simulink library "Tire_MFSwift"  (R2026a)
settings: Solver=VariableStepAuto
undefined symbols (not defined in the file): Left, mfswift_Veh_PARAM, Vehicle, Visual, X, Y, Z
libraries: nesl_utility x24, sm_lib x15, TireBody_Systems x1, mfswift_library x1, mfswift_simscape_library x1, Tire_Utilities x1, $bdroot x1
(part 2 of 2)

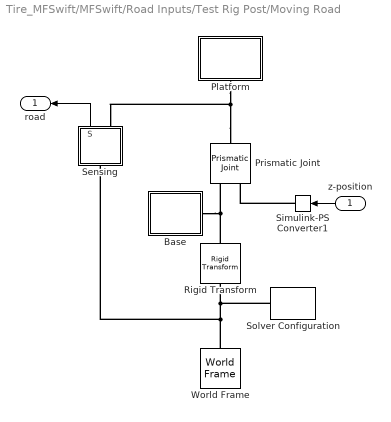
== system Tire_MFSwift/MFSwift/Road Inputs/Test Rig Post/Moving Road ==
  z-position : Inport
  Base : Subsystem
  Platform : Subsystem
  Prismatic Joint : sm_lib/Joints/Prismatic Joint  JointMode=Normal  CompositeWrenchDir=FollowerOnBase  CompositeWrenchFrame=BaseFrame  SenseConstraintForce=off  SenseConstraintTorque=off  SenseTotalForce=off  SenseTotalTorque=off  PositionTargetSpecify=off  PositionTargetPriority=High  PositionTargetValue=0  PositionTargetValueUnits=m  VelocityTargetSpecify=off  VelocityTargetPriority=High  VelocityTargetValue=0  VelocityTargetValueUnits=m/s  EquilibriumPosition=0  EquilibriumPositionUnits=m  SpringStiffness=0  SpringStiffnessUnits=N/m  DampingCoefficient=0  DampingCoefficientUnits=N/(m/s)  LowerLimitSpecify=off  LowerLimitBound=-1  LowerLimitBoundUnits=m  LowerLimitStiffness=1e6  LowerLimitStiffnessUnits=N/m  LowerLimitDamping=1e3  LowerLimitDampingUnits=N/(m/s)  LowerLimitTransitionRegionWidth=1e-4  LowerLimitTransitionRegionWidthUnits=m  UpperLimitSpecify=off  UpperLimitBound=1  UpperLimitBoundUnits=m  UpperLimitStiffness=1e6  UpperLimitStiffnessUnits=N/m  UpperLimitDamping=1e3  UpperLimitDampingUnits=N/(m/s)  UpperLimitTransitionRegionWidth=1e-4  UpperLimitTransitionRegionWidthUnits=m  TorqueActuationMode=ComputedTorque  MotionActuationMode=InputMotion  SensePosition=off  SenseVelocity=off  SenseAcceleration=off  SenseTorqueForce=off  SenseLowerLimitTorqueForce=off  SenseUpperLimitTorqueForce=off
  Rigid Transform : sm_lib/Frames and Transforms/Rigid Transform  RotationMethod=None  FollAlignAxisA=+X  BaseAlignAxisA=+Y  FollAlignAxisB=+Y  BaseAlignAxisB=+Z  RotationStandardAxis=+X  RotationAngle=0  RotationAngleUnits=deg  RotationArbitraryAxis=[0 0 1]  RotationSequenceAxes=FollowerAxes  RotationSequence=XYX  RotationSequenceAngles=[0 0 0]  RotationSequenceAnglesUnits=deg  RotationMatrix=[1 0 0; 0 1 0; 0 0 1]  Quaternion=[1 0 0 0]  TranslationMethod=Cartesian  TranslationCartesianOffset=[mfswift_Veh_PARAM.Body.Length*frontrear mfswift_Veh_PARAM.WheelBase/2*leftright 0]  TranslationCartesianOffsetUnits=m  TranslationStandardAxis=+Z  TranslationStandardOffset=0  TranslationStandardOffsetUnits=m  TranslationROffset=0  TranslationROffsetUnits=m  TranslationThetaOffset=0  TranslationThetaOffsetUnits=deg  TranslationZOffset=0  TranslationZOffsetUnits=m
  Sensing : Subsystem
  Simulink-PS Converter1 : nesl_utility/Simulink-PS Converter  PhysicalDomain=network_engine_domain  SubClassName=ps_input  LeftPortType=input  RightPortType=output  PseudoPeriodic=off  Frequencies=[]  NoiseDistribution=none  NoiseParameters=[]  Unit=1  AffineConversion=off  FilteringAndDerivatives=zero  SimscapeFilterOrder=2  InputFilterTimeConstant=response_time*0.1075  UdotUserProvided=1
  Solver Configuration : nesl_utility/Solver Configuration  PhysicalDomain=network_engine_domain  SubClassName=solver  LeftPortType=input  RightPortType=generic  Tones=[]  Harmonics=[]  SimulateNoise=off  Profile=off  UseLocalSampling=off  EnableSwitchedLinearOptims=on  FrequencyDomain=off  UseCCode=off  RelTol=0.001  AbsTol=1e-06  MinStep=1e-09  ToWorkspace=off  RevertToSquareIcSolve=off  NumHomotopyIterations=100  PhasorMode=off  PhasorModeNumHarmonics=1  ConsistencySolver=NEWTON_FTOL  CanonicalOrdering=UNORDERED  OptimizeIntermediates=UNOPTIMIZED  IndexReductionMethod=DerivativeReplacement  DoDC=off  ResidualTolerance=1e-09  ConsistencyTolSource=GLOBAL  ConsistencyAbsTol=0.001  ConsistencyRelTol=0.001  ConsistencyTolFactor=0.001  UseLocalSolver=off  LocalSolverChoice=NE_BACKWARD_EULER_ADVANCER  ResolveIndetEquations=on  FunctionEvalNumThread=1  LocalSolverSampleTime=0.001  DoFixedCost=off  MaxNonlinIter=3  MaxModeIter=2  ComputeImpulses=off  ImpulseIterations=2  LinearAlgebra=Sparse  LinearAlgebraNumThread=0  EquationFormulation=NE_TIME_EF  DelaysMemoryBudget=1024  AutomaticFiltering=on  FilteringTimeConstant=0.001  PartitionStorageMethod=AS_NEEDED  PartitionMemoryBudget=1024  PartitionMethod=FAST  MultibodyUseLocalSolver=off  MultibodyLocalSolverChoice=ODE1  MultibodyLocalSolverSampleTime=0.001
  World Frame : sm_lib/Frames and Transforms/World Frame
  road : Outport
  wires:
  Sensing/1(S) -> road/1
  z-position/1 -> Simulink-PS Converter1/1
  connections:
  Prismatic Joint/RConn1 -- Sensing/RConn1 -- Platform/LConn1
  Prismatic Joint/LConn1 -- Base/RConn1 -- Rigid Transform/RConn1
  Sensing/LConn1 -- Solver Configuration/RConn1 -- Rigid Transform/LConn1 -- World Frame/RConn1
  Simulink-PS Converter1/RConn1 -- Prismatic Joint/LConn2

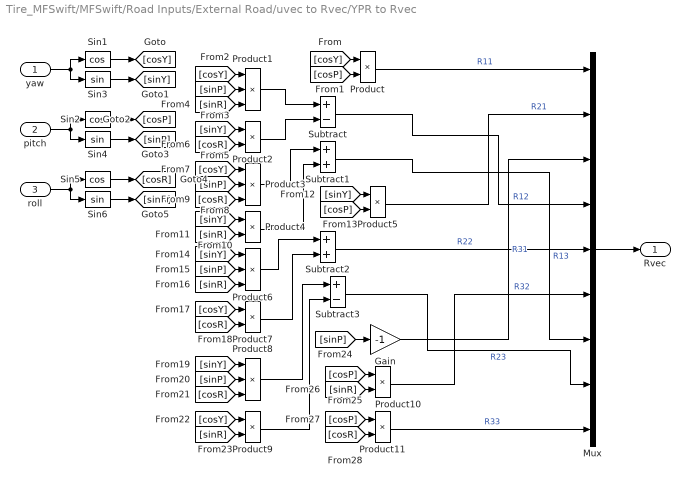
== system Tire_MFSwift/MFSwift/Road Inputs/External Road/uvec to Rvec/YPR to Rvec ==
  yaw : Inport
  pitch : Inport  Port=2
  roll : Inport  Port=3
  Gain : Gain  Gain=-1
  Mux : Mux  Inputs=9
  Product{,2,4..5,7,9..11} (8 alike) : Product
  Product{1,3,6,8} (4 alike) : Product  Inputs=3
  Sin1 : Trigonometry  Operator=cos
  Sin2 : Trigonometry  Operator=cos
  Sin3 : Trigonometry
  Sin4 : Trigonometry
  Sin5 : Trigonometry  Operator=cos
  Sin6 : Trigonometry
  Subtract : Sum  Inputs=+-
  Subtract1 : Sum
  Subtract2 : Sum
  Subtract3 : Sum  Inputs=+-
  Rvec : Outport
  wires:
  Sin4/1 -> [sinP]
  [sinP] -> Product6/2
  Product4/1 -> Subtract1/2
  [cosY] -> Product3/1
  Subtract3/1 -> Mux/8  "R23"
  [sinY] -> Product8/1
  Subtract2/1 -> Mux/5  "R22"
  [cosP] -> Product10/1
  [cosY] -> Product/1
  [sinP] -> Product3/2
  [sinY] -> Product2/1
  yaw/1 -> Sin1/1, Sin3/1
  Subtract/1 -> Mux/4  "R12"
  Sin2/1 -> [cosP]
  Sin5/1 -> [cosR]
  [cosR] -> Product11/2
  [sinP] -> Gain/1
  [sinR] -> Product10/2
  [sinR] -> Product1/3
  [cosR] -> Product8/3
  roll/1 -> Sin5/1, Sin6/1
  Product5/1 -> Mux/2  "R21"
  Product8/1 -> Subtract3/1
  Sin1/1 -> [cosY]
  [cosR] -> Product7/2
  Product11/1 -> Mux/9  "R33"
  Product1/1 -> Subtract/1
  [sinY] -> Product4/1
  [sinP] -> Product8/2
  [cosY] -> Product1/1
  [cosY] -> Product7/1
  Sin6/1 -> [sinR]
  Product2/1 -> Subtract/2
  [cosY] -> Product9/1
  [cosP] -> Product11/1
  [cosP] -> Product/2
  Product9/1 -> Subtract3/2
  [cosR] -> Product2/2
  [sinR] -> Product4/2
  Product/1 -> Mux/1  "R11"
  [sinY] -> Product5/1
  Product7/1 -> Subtract2/2
  [cosP] -> Product5/2
  Sin3/1 -> [sinY]
  Product10/1 -> Mux/6  "R32"
  [sinP] -> Product1/2
  [cosR] -> Product3/3
  Gain/1 -> Mux/3  "R31"
  Mux/1 -> Rvec/1
  pitch/1 -> Sin4/1, Sin2/1
  [sinY] -> Product6/1
  Subtract1/1 -> Mux/7  "R13"
  Product6/1 -> Subtract2/1
  [sinR] -> Product6/3
  [sinR] -> Product9/2
  Product3/1 -> Subtract1/1

== system Tire_MFSwift/MFSwift/Road Inputs/Test Rig Post/Moving Road/Base ==
  Platform1 : sm_lib/Body Elements/Cylindrical Solid  CylinderRadius=0.15  CylinderRadiusUnits=m  CylinderLength=0.5  CylinderLengthUnits=m  ExportEntireGeometry=off  InertiaType=CalculateFromGeometry  BasedOnType=Density  Density=1000  DensityUnits=kg/(m^3)  Mass=1  MassUnits=kg  CenterOfMass=[0 0 0]  CenterOfMassUnits=m  MomentsOfInertia=[1 1 1]  MomentsOfInertiaUnits=kg*m^2  ProductsOfInertia=[0 0 0]  ProductsOfInertiaUnits=kg*m^2  GraphicType=FromGeometry  MarkerShape=Sphere  MarkerSize=10  GraphicVisPropType=SimpleVisualProperties  GraphicDiffuseColor=[0.5 0.5 0.5]  GraphicOpacity=0.5  GraphicSpecularColor=[0.5 0.5 0.5 1.0]  GraphicAmbientColor=[0.15 0.15 0.15 1.0]  GraphicEmissiveColor=[0.0 0.0 0.0 1.0]  GraphicShininess=75  DoExposeReferenceFrame=on  SerializedFrames=<Frames/>
  Rigid Transform1 : sm_lib/Frames and Transforms/Rigid Transform  RotationMethod=None  FollAlignAxisA=+X  BaseAlignAxisA=+Y  FollAlignAxisB=+Y  BaseAlignAxisB=+Z  RotationStandardAxis=+Z  RotationAngle=0  RotationAngleUnits=deg  RotationArbitraryAxis=[0 0 1]  RotationSequenceAxes=FollowerAxes  RotationSequence=XYX  RotationSequenceAngles=[0 0 0]  RotationSequenceAnglesUnits=deg  RotationMatrix=[1 0 0; 0 1 0; 0 0 1]  Quaternion=[1 0 0 0]  TranslationMethod=Cartesian  TranslationCartesianOffset=[0 0 -0.50]  TranslationCartesianOffsetUnits=m  TranslationStandardAxis=+Z  TranslationStandardOffset=0  TranslationStandardOffsetUnits=m  TranslationROffset=0  TranslationROffsetUnits=m  TranslationThetaOffset=0  TranslationThetaOffsetUnits=deg  TranslationZOffset=0  TranslationZOffsetUnits=m
  B : PMIOPort  Side=Right
  connections:
  Rigid Transform1/RConn1 -- Platform1/RConn1
  Rigid Transform1/LConn1 -- B/RConn1

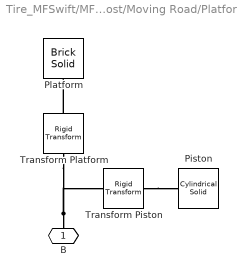
== system Tire_MFSwift/MFSwift/Road Inputs/Test Rig Post/Moving Road/Platform ==
  Piston : sm_lib/Body Elements/Cylindrical Solid  CylinderRadius=0.07  CylinderRadiusUnits=m  CylinderLength=0.4  CylinderLengthUnits=m  ExportEntireGeometry=off  InertiaType=CalculateFromGeometry  BasedOnType=Density  Density=1000  DensityUnits=kg/(m^3)  Mass=1  MassUnits=kg  CenterOfMass=[0 0 0]  CenterOfMassUnits=m  MomentsOfInertia=[1 1 1]  MomentsOfInertiaUnits=kg*m^2  ProductsOfInertia=[0 0 0]  ProductsOfInertiaUnits=kg*m^2  GraphicType=FromGeometry  MarkerShape=Sphere  MarkerSize=10  GraphicVisPropType=SimpleVisualProperties  GraphicDiffuseColor=[0.8 0.8 0.8]  GraphicOpacity=1.0  GraphicSpecularColor=[0.5 0.5 0.5 1.0]  GraphicAmbientColor=[0.15 0.15 0.15 1.0]  GraphicEmissiveColor=[0.0 0.0 0.0 1.0]  GraphicShininess=75  DoExposeReferenceFrame=on  SerializedFrames=<Frames/>
  Platform : sm_lib/Body Elements/Brick Solid  BrickDimensions=[0.5 0.5 0.04]  BrickDimensionsUnits=m  ExportEntireGeometry=off  InertiaType=CalculateFromGeometry  BasedOnType=Density  Density=1000  DensityUnits=kg/(m^3)  Mass=1  MassUnits=kg  CenterOfMass=[0 0 0]  CenterOfMassUnits=m  MomentsOfInertia=[1 1 1]  MomentsOfInertiaUnits=kg*m^2  ProductsOfInertia=[0 0 0]  ProductsOfInertiaUnits=kg*m^2  GraphicType=FromGeometry  MarkerShape=Sphere  MarkerSize=10  GraphicVisPropType=SimpleVisualProperties  GraphicDiffuseColor=[0.5 0.5 0.5]  GraphicOpacity=1.0  GraphicSpecularColor=[0.5 0.5 0.5 1.0]  GraphicAmbientColor=[0.15 0.15 0.15 1.0]  GraphicEmissiveColor=[0.0 0.0 0.0 1.0]  GraphicShininess=75  DoExposeReferenceFrame=on  SerializedFrames=<Frames/>
  Transform Piston : sm_lib/Frames and Transforms/Rigid Transform  RotationMethod=None  FollAlignAxisA=+X  BaseAlignAxisA=+Y  FollAlignAxisB=+Y  BaseAlignAxisB=+Z  RotationStandardAxis=+Z  RotationAngle=0  RotationAngleUnits=deg  RotationArbitraryAxis=[0 0 1]  RotationSequenceAxes=FollowerAxes  RotationSequence=XYX  RotationSequenceAngles=[0 0 0]  RotationSequenceAnglesUnits=deg  RotationMatrix=[1 0 0; 0 1 0; 0 0 1]  Quaternion=[1 0 0 0]  TranslationMethod=Cartesian  TranslationCartesianOffset=[0 0 -0.26]  TranslationCartesianOffsetUnits=m  TranslationStandardAxis=+Z  TranslationStandardOffset=0  TranslationStandardOffsetUnits=m  TranslationROffset=0  TranslationROffsetUnits=m  TranslationThetaOffset=0  TranslationThetaOffsetUnits=deg  TranslationZOffset=0  TranslationZOffsetUnits=m
  Transform Platform : sm_lib/Frames and Transforms/Rigid Transform  RotationMethod=None  FollAlignAxisA=+X  BaseAlignAxisA=+Y  FollAlignAxisB=+Y  BaseAlignAxisB=+Z  RotationStandardAxis=+Z  RotationAngle=0  RotationAngleUnits=deg  RotationArbitraryAxis=[0 0 1]  RotationSequenceAxes=FollowerAxes  RotationSequence=XYX  RotationSequenceAngles=[0 0 0]  RotationSequenceAnglesUnits=deg  RotationMatrix=[1 0 0; 0 1 0; 0 0 1]  Quaternion=[1 0 0 0]  TranslationMethod=Cartesian  TranslationCartesianOffset=[0 0 -0.06]  TranslationCartesianOffsetUnits=m  TranslationStandardAxis=+Z  TranslationStandardOffset=0  TranslationStandardOffsetUnits=m  TranslationROffset=0  TranslationROffsetUnits=m  TranslationThetaOffset=0  TranslationThetaOffsetUnits=deg  TranslationZOffset=0  TranslationZOffsetUnits=m
  B : PMIOPort  Side=Left
  connections:
  B/RConn1 -- Transform Piston/LConn1 -- Transform Platform/LConn1
  Transform Platform/RConn1 -- Platform/RConn1
  Transform Piston/RConn1 -- Piston/RConn1

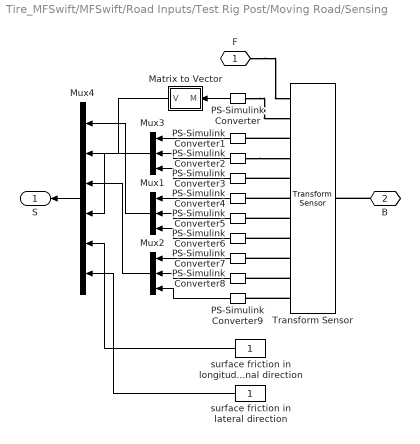
== system Tire_MFSwift/MFSwift/Road Inputs/Test Rig Post/Moving Road/Sensing ==
  Matrix to Vector : Subsystem
  Mux1 : Mux  Inputs=3
  Mux2 : Mux  Inputs=3
  Mux3 : Mux  Inputs=3
  Mux4 : Mux  Inputs=6
  PS-Simulink Converter{,1..9} (10 alike) : nesl_utility/PS-Simulink Converter  PhysicalDomain=network_engine_domain  SubClassName=ps_output  LeftPortType=input  RightPortType=output  PseudoPeriodic=off  Frequencies=[]  VectorFormat=1-D array  Unit=1  AffineConversion=off
  Transform Sensor : sm_lib/Frames and Transforms/Transform Sensor  MeasurementFrame=World  RotationSequence=XYX  SenseAngle=off  SenseAxis=off  SenseQ=off  SenseR=on  SenseRotationSequence=off  SenseOmegaX=on  SenseOmegaY=on  SenseOmegaZ=on  SenseOmega=off  SenseQDot=off  SenseRDot=off  SenseRotationSequenceDot=off  SenseAlphaX=off  SenseAlphaY=off  SenseAlphaZ=off  SenseAlpha=off  SenseQDDot=off  SenseRDDot=off  SenseX=on  SenseY=on  SenseZ=on  SenseXYZ=off  SenseRad=off  SenseAzim=off  SenseDist=off  SenseInc=off  SenseXDot=on  SenseYDot=on  SenseZDot=on  SenseXYZDot=off  SenseRadDot=off  SenseAzimDot=off  SenseDistDot=off  SenseIncDot=off  SenseXDDot=off  SenseYDDot=off  SenseZDDot=off  SenseXYZDDot=off  SenseRadDDot=off  SenseAzimDDot=off  SenseDistDDot=off  SenseIncDDot=off
  surface friction in lateral direction : Constant
  surface friction in longitudinal direction : Constant
  F : PMIOPort  Side=Right
  B : PMIOPort  Port=2  Side=Left
  S : Outport
  wires:
  surface friction in lateral direction/1 -> Mux4/6
  surface friction in longitudinal direction/1 -> Mux4/5
  Matrix to Vector/1(V) -> Mux4/2
  PS-Simulink Converter8/1 -> Mux2/2
  PS-Simulink Converter1/1 -> Mux3/1
  Mux3/1 -> Mux4/4
  PS-Simulink Converter9/1 -> Mux2/3
  Mux1/1 -> Mux4/1
  Mux2/1 -> Mux4/3
  Mux4/1 -> S/1
  PS-Simulink Converter3/1 -> Mux3/3
  PS-Simulink Converter/1 -> Matrix to Vector/1(M)
  PS-Simulink Converter6/1 -> Mux1/3
  PS-Simulink Converter4/1 -> Mux1/1
  PS-Simulink Converter7/1 -> Mux2/1
  PS-Simulink Converter5/1 -> Mux1/2
  PS-Simulink Converter2/1 -> Mux3/2
  connections:
  Transform Sensor/RConn5 -- PS-Simulink Converter3/LConn1
  Transform Sensor/RConn6 -- PS-Simulink Converter4/LConn1
  Transform Sensor/RConn10 -- PS-Simulink Converter8/LConn1
  Transform Sensor/RConn3 -- PS-Simulink Converter1/LConn1
  Transform Sensor/RConn11 -- PS-Simulink Converter9/LConn1
  Transform Sensor/RConn8 -- PS-Simulink Converter6/LConn1
  Transform Sensor/RConn7 -- PS-Simulink Converter5/LConn1
  PS-Simulink Converter/LConn1 -- Transform Sensor/RConn2
  Transform Sensor/RConn9 -- PS-Simulink Converter7/LConn1
  PS-Simulink Converter2/LConn1 -- Transform Sensor/RConn4
  F/RConn1 -- Transform Sensor/RConn1
  B/RConn1 -- Transform Sensor/LConn1

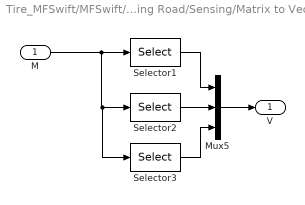
== system Tire_MFSwift/MFSwift/Road Inputs/Test Rig Post/Moving Road/Sensing/Matrix to Vector ==
  M : Inport
  Mux5 : Mux  Inputs=3
  Selector1 : Selector  NumberOfDimensions=2  InputPortWidth=9  IndexOptions=Index vector (dialog),Index vector (dialog)  Indices=[1 2 3],1  OutputSizes=1,1
  Selector2 : Selector  NumberOfDimensions=2  InputPortWidth=9  IndexOptions=Index vector (dialog),Index vector (dialog)  Indices=[1 2 3],2  OutputSizes=1,1
  Selector3 : Selector  NumberOfDimensions=2  InputPortWidth=9  IndexOptions=Index vector (dialog),Index vector (dialog)  Indices=[1 2 3],3  OutputSizes=1,1
  V : Outport
  wires:
  Selector1/1 -> Mux5/1
  Mux5/1 -> V/1
  M/1 -> Selector1/1, Selector2/1, Selector3/1
  Selector3/1 -> Mux5/3
  Selector2/1 -> Mux5/2
